simulink model "sf_cruise_control"  (Simulink 7.6)
settings: Solver=ode5  SolverMode=SingleTasking  StartTime=0.0  StopTime=inf  FixedStep=0.005  RelTol=1e-3
model workspace (MAT data in the model file):
  Kd = 30
  Ki = 10
  Kp = 30
  set_speed : Simulink.Signal (value not decoded)
  target_speed : Simulink.Signal (value not decoded)
values from neighbouring files (symbols this model uses):
  Ki = 253080    [sf_electrohydraulic_data.m]
undefined symbols (not defined in the file or in its folder): DiscIntNeverNeededParam
libraries: simulink x1
settings Model: Creator=The MathWorks Inc.  CovMetricSettings=dcmtr  CovHTMLOptions=-aTS=0 -bRG=1 -bTC=0 -hTR=0 -nFC=1  ExtModeAutoUpdateStatusClock=off
settings OptimizationCC: BooleanDataType=off  InlineInvariantSignals=on  InitFltsAndDblsToZero=on  EfficientMapNaN2IntZero=off
settings DebuggingCC: SaveWithParameterizedLinksMsg=none  SignalResolutionControl=TryResolveAllWithWarning  SolverPrmCheckMsg=none  MultiTaskDSMMsg=warning  MultiTaskCondExecSysMsg=none  StrictBusMsg=None
settings HardwareCC: TargetEndianess=LittleEndian  TargetHWDeviceType=MATLAB Host  ProdEqTarget=off
settings SFSimCC: SimParseCustomCode=off
settings RTWCC: GenerateReport=on  LaunchReport=on  IncludeERTFirstTime=on
settings GRTTargetCC: TargetFcnLib=ansi_tfl_tmw.mat

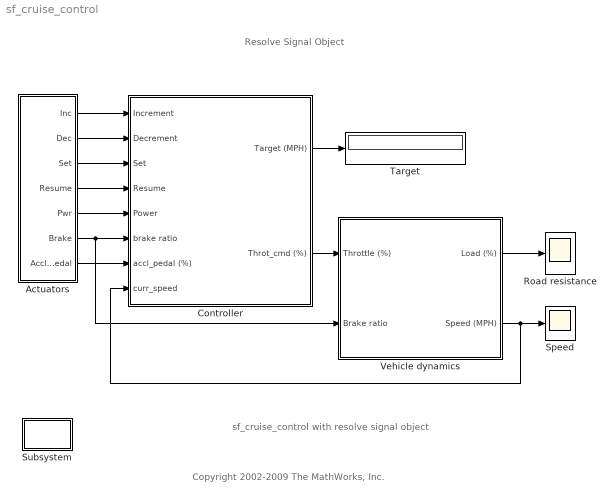
== system sf_cruise_control ==
  note: sf_cruise_control with resolve signal object
  note: Resolve Signal Object
  note: Copyright 2002-2009 The MathWorks, Inc.
  Actuators : Subsystem
      mask Display: disp('Actuator \n Signals')
  Controller : Subsystem
  Road resistance : Scope
      settings: TimeRange=80  YMin=-10  YMax=40  SampleInput=on  SampleTime=0.5
  Speed : Scope
      settings: TickLabels=on  TimeRange=80  YMin=-20  YMax=100  SampleInput=on  SampleTime=0.5
  Subsystem : Subsystem
      mask Display: disp('Info')
  Target : Display
  Vehicle dynamics : Subsystem
  wires:
  Actuators/3(Set) -> Controller/3(Set)
  Actuators/4(Resume) -> Controller/4(Resume)
  Actuators/5(Pwr) -> Controller/5(Power)
  Actuators/6(Brake) -> Vehicle dynamics/2(Brake ratio), Controller/6(brake ratio)
  Actuators/7(Accl_pedal) -> Controller/7(accl_pedal (%))
  Controller/2(Throt_cmd (%)) -> Vehicle dynamics/1(Throttle (%))
  Vehicle dynamics/2(Speed (MPH)) -> Speed/1, Controller/8(curr_speed)
  Controller/1(Target (MPH)) -> Target/1
  Actuators/1(Inc) -> Controller/1(Increment)
  Actuators/2(Dec) -> Controller/2(Decrement)
  Vehicle dynamics/1(Load (%)) -> Road resistance/1

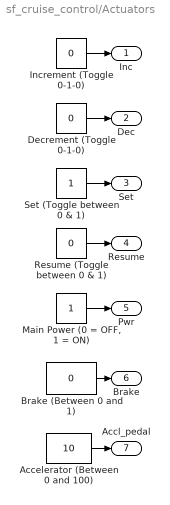
== system sf_cruise_control/Actuators ==
  Accelerator (Between 0 and 100) : Constant  Value=10
  Brake (Between 0 and 1) : Constant  Value=0
  Decrement (Toggle 0-1-0) : Constant  Value=0
  Increment (Toggle 0-1-0) : Constant  Value=0
  "Main Power (0 = OFF, 1 = ON)" : Constant
  Resume (Toggle between 0 & 1) : Constant  Value=0
  Set (Toggle between 0 & 1) : Constant
  Inc : Outport
  Dec : Outport  Port=2
  Set : Outport  Port=3
  Resume : Outport  Port=4
  Pwr : Outport  Port=5
  Brake : Outport  Port=6
  Accl_pedal : Outport  Port=7
  wires:
  Increment (Toggle 0-1-0)/1 -> Inc/1
  Decrement (Toggle 0-1-0)/1 -> Dec/1
  Set (Toggle between 0 & 1)/1 -> Set/1
  Resume (Toggle between 0 & 1)/1 -> Resume/1
  "Main Power (0 = OFF, 1 = ON)"/1 -> Pwr/1
  Brake (Between 0 and 1)/1 -> Brake/1
  Accelerator (Between 0 and 100)/1 -> Accl_pedal/1

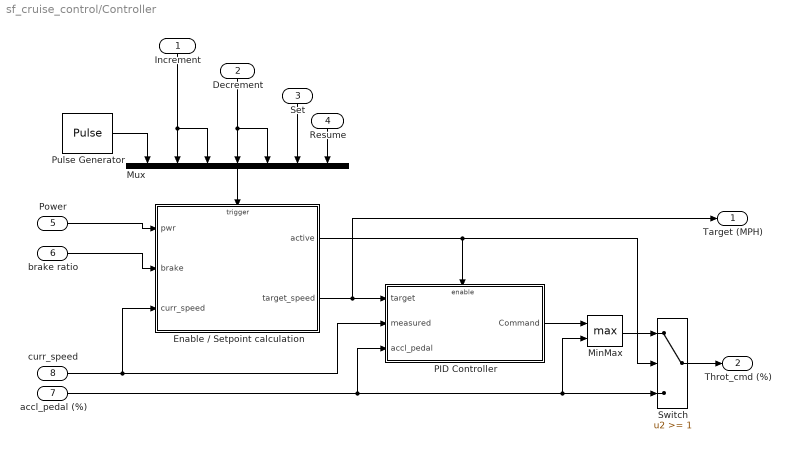
== system sf_cruise_control/Controller ==
  Increment : Inport
  Decrement : Inport  Port=2
  Set : Inport  Port=3
  Resume : Inport  Port=4
  Power : Inport  Port=5
  brake ratio : Inport  Port=6
  accl_pedal (%) : Inport  Port=7
  curr_speed : Inport  Port=8
  Enable / Setpoint calculation : Stateflow chart  TreatAsAtomicUnit=on
  MinMax : MinMax  Function=max  Inputs=2  ZeroCross=off  SaturateOnIntegerOverflow=on  InputSameDT=on
  Mux : Mux  Inputs=7
  PID Controller : Subsystem  TreatAsAtomicUnit=on
  Pulse Generator : DiscretePulseGenerator  SampleTime=.05
  Switch : Switch  Threshold=1  ZeroCross=off  InputSameDT=on
  Target (MPH) : Outport
  Throt_cmd (%) : Outport  Port=2
  wires:
  Pulse Generator/1 -> Mux/1
  PID Controller/1(Command) -> MinMax/1
  MinMax/1 -> Switch/1
  Enable / Setpoint calculation/1(active) -> PID Controller/Enable, Switch/2
  Switch/1 -> Throt_cmd (%)/1
  brake ratio/1 -> Enable / Setpoint calculation/2(brake)
  Power/1 -> Enable / Setpoint calculation/1(pwr)
  Resume/1 -> Mux/7
  Set/1 -> Mux/6
  Decrement/1 -> Mux/4, Mux/5
  Increment/1 -> Mux/2, Mux/3
  accl_pedal (%)/1 -> MinMax/2, Switch/3, PID Controller/3(accl_pedal)
  curr_speed/1 -> Enable / Setpoint calculation/3(curr_speed), PID Controller/2(measured)
  Enable / Setpoint calculation/2(target_speed) -> Target (MPH)/1, PID Controller/1(target)
  Mux/1 -> Enable / Setpoint calculation/Trigger

== system sf_cruise_control/Subsystem ==
  note: This model was discussed in:
      |
      | Aldrich, W. "Coverage Analysis for Model Based Design Tool",
      | Proceedings, 18th Testing Computer Software Conference, June 2001
      |
      | Available for download from
      | http://www.mathworks.com/products/simulink/technicalliterature.shtml

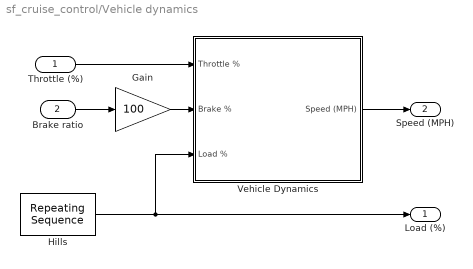
== system sf_cruise_control/Vehicle dynamics ==
  Throttle (%) : Inport
  Brake ratio : Inport  Port=2
  Gain : Gain  Gain=100  SaturateOnIntegerOverflow=on  OutDataTypeStr=Inherit: Same as input  ParamDataTypeStr=Inherit: Same as input
  Hills : simulink/Sources/Repeating Sequence  SystemSampleTime=-1  rep_seq_t=[0 2 3 5 6 8]*10  rep_seq_y=[10 15 5 20 10 -2]
  Vehicle Dynamics : Subsystem
  Load (%) : Outport
  Speed (MPH) : Outport  Port=2
  wires:
  Hills/1 -> Load (%)/1, Vehicle Dynamics/3(Load %)
  Brake ratio/1 -> Gain/1
  Throttle (%)/1 -> Vehicle Dynamics/1(Throttle %)
  Vehicle Dynamics/1(Speed (MPH)) -> Speed (MPH)/1
  Gain/1 -> Vehicle Dynamics/2(Brake %)

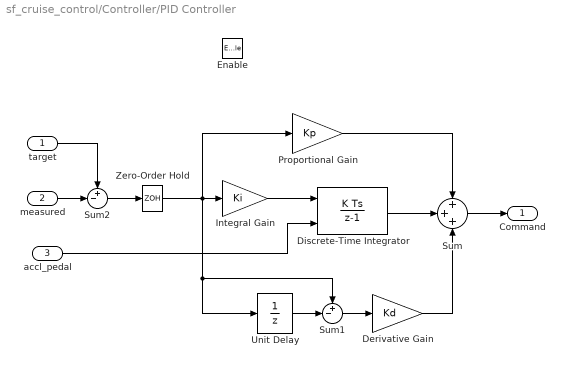
== system sf_cruise_control/Controller/PID Controller ==
  target : Inport
  measured : Inport  Port=2
  accl_pedal : Inport  Port=3
  Enable : EnablePort  StatesWhenEnabling=reset  ZeroCross=off
  Derivative Gain : Gain  Gain=Kd  SaturateOnIntegerOverflow=on  OutDataTypeStr=Inherit: Same as input  ParamDataTypeStr=Inherit: Same as input
  Discrete-Time Integrator : DiscreteIntegrator  InitialConditionSource=external  SampleTime=0.1  UpperSaturationLimit=20  LowerSaturationLimit=-20  ICPrevOutput=DiscIntNeverNeededParam  ICPrevScaledInput=DiscIntNeverNeededParam
  Integral Gain : Gain  Gain=Ki  SaturateOnIntegerOverflow=on  OutDataTypeStr=Inherit: Same as input  ParamDataTypeStr=Inherit: Same as input
  Proportional Gain : Gain  Gain=Kp  SaturateOnIntegerOverflow=on  OutDataTypeStr=Inherit: Same as input  ParamDataTypeStr=Inherit: Same as input
  Sum : Sum  Inputs=+++  SaturateOnIntegerOverflow=on  InputSameDT=on  OutDataTypeStr=Inherit: Same as first input
  Sum1 : Sum  Inputs=+-|  SaturateOnIntegerOverflow=on  InputSameDT=on  OutDataTypeStr=Inherit: Same as first input
  Sum2 : Sum  Inputs=+-|  SaturateOnIntegerOverflow=on  InputSameDT=on  OutDataTypeStr=Inherit: Same as first input
  Unit Delay : UnitDelay  SampleTime=0.1
  Zero-Order Hold : ZeroOrderHold  SampleTime=0.1
  Command : Outport
  wires:
  Zero-Order Hold/1 -> Integral Gain/1, Sum1/1, Unit Delay/1, Proportional Gain/1
  accl_pedal/1 -> Discrete-Time Integrator/2
  Integral Gain/1 -> Discrete-Time Integrator/1
  measured/1 -> Sum2/2
  target/1 -> Sum2/1
  Sum/1 -> Command/1
  Sum2/1 -> Zero-Order Hold/1
  Proportional Gain/1 -> Sum/1
  Derivative Gain/1 -> Sum/3
  Discrete-Time Integrator/1 -> Sum/2
  Sum1/1 -> Derivative Gain/1
  Unit Delay/1 -> Sum1/2

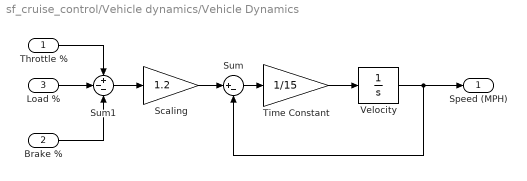
== system sf_cruise_control/Vehicle dynamics/Vehicle Dynamics ==
  Throttle % : Inport
  Brake % : Inport  Port=2
  Load % : Inport  Port=3
  Scaling : Gain  Gain=1.2  SaturateOnIntegerOverflow=on  OutDataTypeStr=Inherit: Same as input  ParamDataTypeStr=Inherit: Same as input
  Sum : Sum  Inputs=|+-  SaturateOnIntegerOverflow=on  InputSameDT=on  OutDataTypeStr=Inherit: Same as first input
  Sum1 : Sum  Inputs=+--  SaturateOnIntegerOverflow=on  InputSameDT=on  OutDataTypeStr=Inherit: Same as first input
  Time Constant : Gain  Gain=1/15  SaturateOnIntegerOverflow=on  OutDataTypeStr=Inherit: Same as input  ParamDataTypeStr=Inherit: Same as input
  Velocity : Integrator  LimitOutput=on  LowerSaturationLimit=0  ZeroCross=off
  Speed (MPH) : Outport
  wires:
  Time Constant/1 -> Velocity/1
  Sum/1 -> Time Constant/1
  Scaling/1 -> Sum/1
  Sum1/1 -> Scaling/1
  Velocity/1 -> Speed (MPH)/1, Sum/2
  Load %/1 -> Sum1/2
  Throttle %/1 -> Sum1/1
  Brake %/1 -> Sum1/3

== stateflow chart Controller/Enable / Setpoint calculation ==
  state Set_Point_Calculation [parallel]
    settings: executionOrder=1
    state Hold
      Hold -> (junction 13) [order 1] : Set [pwr]
          | {
          | target_speed = curr_speed;
          | set_speed = curr_speed;
          | }
      Hold -> (junction 14) [order 2] : Resume [pwr]
      (junction 14) -> (junction 15) [order 2]
      (junction 14) -> (junction 15) [order 1] : [set_speed > 0]
          |
          | {target_speed = ...
          | set_speed;}
    state Increment
      en: target_speed++;
      Increment -> Increment [order 1] : every(10,Update)
          | {target_speed++;}
    state Decrement
      en: target_speed--;
      Decrement -> Decrement [order 1] : every(10,Update)
          | {target_speed--;}
    (default) -> Hold
    Hold -> Increment [order 2] : INC_BD
        | [in(Enable.on.active)]
    Increment -> Hold [order 1] : INC_BU
    Decrement -> Hold [order 1] : DEC_BU
    Hold -> Decrement [order 1] : DEC_BD
        | [in(Enable.on.active)]
  state Enable [parallel]
    settings: executionOrder=2
    state Off
    state on
      state active
      state overide
        target_speed = 0;
      state no_target
      no_target -> active : Set
      (default) -> no_target
      active -> overide : [brake]
      overide -> active : Set | Resume
    on -> Off : [!pwr]
    Off -> on : [pwr]
    (default) -> Off
  data: pwr input boolean; brake input boolean; active output unknown; target_speed output double; set_speed local double; curr_speed input double
  events: Update input RISING_EDGE_EVENT; INC_BD input RISING_EDGE_EVENT; INC_BU input FALLING_EDGE_EVENT; DEC_BD input RISING_EDGE_EVENT; DEC_BU input FALLING_EDGE_EVENT; Set input EITHER_EDGE_EVENT; Resume input EITHER_EDGE_EVENT
